simulink model "Pt_Engine_TC_CS8"  (Simulink 7.0)
settings: Solver=ode45  StartTime=0  StopTime=20  FixedStep=TSTEP  RelTol=1e-3
PreLoadFcn:
  | cd extensions\simulink\pt_engine_tc
  | mengine_carpet_eclass
  | torq_conv_map_eclass
  | Run_ft4wd_eclass
  | cd ..\..\..
undefined symbols (not defined in the file): AV_ENG_IDLE, IENG, INV_CAP_TC_TABLE, ITC_INPUT_SHAFT, MENGINE_CARPET, RM_TC_TABLE
libraries: Solver_SF x1
settings Model: Creator=dhall  LastModifiedBy=ywata  ExtModeTrigMode=oneshot  ExtModeArmWhenConnect=off
settings DataIOCC: LimitDataPoints=off  SaveOutput=off  SaveTime=off  SignalLoggingName=sigsOut
settings OptimizationCC: BooleanDataType=off
settings DebuggingCC: SaveWithParameterizedLinksMsg=none  SignalResolutionControl=TryResolveAllWithWarning  SolverPrmCheckMsg=none  MultiTaskDSMMsg=warning  MultiTaskCondExecSysMsg=none  StrictBusMsg=None
settings HardwareCC: TargetUnknown=on
settings RTWCC: IncludeERTFirstTime=on
settings GRTTargetCC: TargetFcnLib=ansi_tfl_tmw.mat  ModelReferenceCompliant=off  MatFileLogging=off

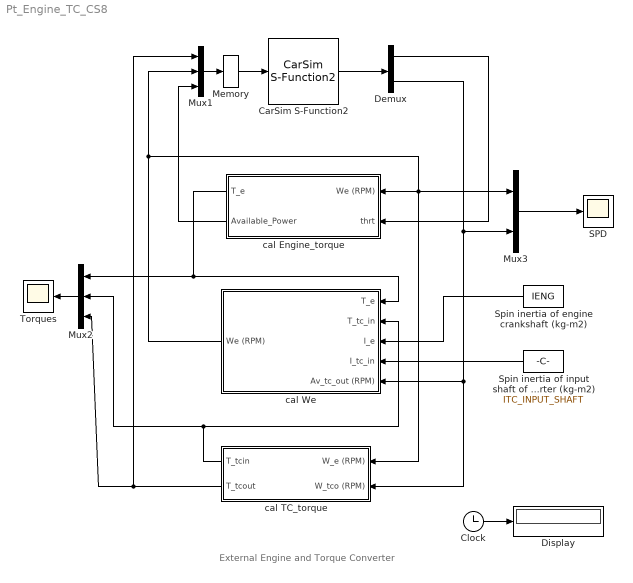
== system Pt_Engine_TC_CS8 ==
  note: External Engine and Torque Converter
  CarSim S-Function2 : Solver_SF/CarSim S-Function2  Priority=1  VehicleCode=???
      settings: AttributesFormatString=Vehicle Code: %<VehicleCode>
  Clock : Clock
      settings: Decimation=10
  Demux : Demux  Outputs=2
  Display : Display
  Memory : Memory
  Mux1 : Mux  Inputs=3
  Mux2 : Mux  Orientation=left  Inputs=3
  Mux3 : Mux  Inputs=2
  SPD : Scope
      settings: TimeRange=20  YMin=0  YMax=4500
  Spin inertia of engine crankshaft (kg-m2) : Constant  Orientation=left  Value=IENG  OutDataType=sfix(16)  OutScaling=2^0
  Spin inertia of input shaft of torque converter (kg-m2) : Constant  Orientation=left  Value=ITC_INPUT_SHAFT  OutDataType=sfix(16)  OutScaling=2^0
  Torques : Scope
      settings: TimeRange=20  YMin=-50  YMax=600
  cal Engine_torque : Subsystem  Orientation=left
  cal TC_torque : Subsystem  Orientation=left
  cal We : Subsystem  Orientation=left
  wires:
  cal We/1(We (RPM)) -> cal TC_torque/1(W_e (RPM)), Mux3/1, cal Engine_torque/1(We (RPM)), Mux1/2
  Spin inertia of engine crankshaft (kg-m2)/1 -> cal We/3(I_e)
  Spin inertia of input shaft of torque converter (kg-m2)/1 -> cal We/4(I_tc_in)
  cal Engine_torque/1(T_e) -> Mux2/1, cal We/1(T_e)
  cal TC_torque/1(T_tcin) -> Mux2/2, cal We/2(T_tc_in)
  CarSim S-Function2/1 -> Demux/1
  Demux/1 -> cal Engine_torque/2(thrt)
  Demux/2 -> cal TC_torque/2(W_tco (RPM)), cal We/5(Av_tc_out (RPM)), Mux3/2
  cal TC_torque/2(T_tcout) -> Mux2/3, Mux1/1
  Mux2/1 -> Torques/1
  Mux3/1 -> SPD/1
  Clock/1 -> Display/1
  cal Engine_torque/2(Available_Power) -> Mux1/3
  Mux1/1 -> Memory/1
  Memory/1 -> CarSim S-Function2/1

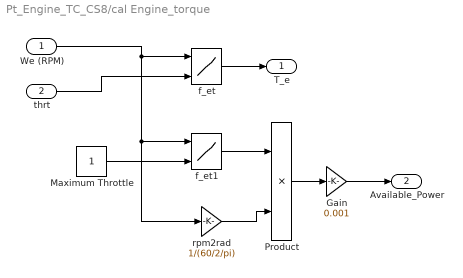
== system Pt_Engine_TC_CS8/cal Engine_torque ==
  We (RPM) : Inport  OutDataType=sfix(16)  OutScaling=2^0
  thrt : Inport  Port=2  OutDataType=sfix(16)  OutScaling=2^0
  Gain : Gain  Gain=0.001  ParameterDataType=sfix(16)  ParameterScaling=2^0  OutDataType=sfix(16)  OutScaling=2^0  SaturateOnIntegerOverflow=on
  Maximum Throttle : Constant  OutDataType=sfix(16)  OutScaling=2^0
  Product : Product  OutDataType=sfix(16)  OutScaling=2^0  SaturateOnIntegerOverflow=on  InputSameDT=on
  f_et : Lookup2D  RowIndex=MENGINE_CARPET(2:19,1)  ColumnIndex=MENGINE_CARPET(1,2:11)  Table=MENGINE_CARPET(2:19,2:11)  OutDataType=sfix(16)  OutScaling=2^0  SaturateOnIntegerOverflow=on  InputSameDT=on
  f_et1 : Lookup2D  RowIndex=MENGINE_CARPET(2:19,1)  ColumnIndex=MENGINE_CARPET(1,2:11)  Table=MENGINE_CARPET(2:19,2:11)  OutDataType=sfix(16)  OutScaling=2^0  SaturateOnIntegerOverflow=on  InputSameDT=on
  rpm2rad : Gain  Gain=1/(60/2/pi)  ParameterDataType=sfix(16)  ParameterScaling=2^0  OutDataType=sfix(16)  OutScaling=2^0  SaturateOnIntegerOverflow=on
  T_e : Outport
  Available_Power : Outport  Port=2
  wires:
  We (RPM)/1 -> f_et/1, rpm2rad/1, f_et1/1
  f_et/1 -> T_e/1
  thrt/1 -> f_et/2
  Maximum Throttle/1 -> f_et1/2
  f_et1/1 -> Product/1
  rpm2rad/1 -> Product/2
  Product/1 -> Gain/1
  Gain/1 -> Available_Power/1

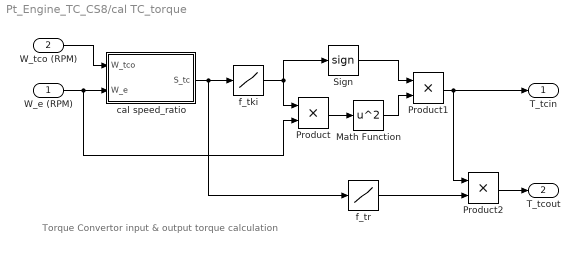
== system Pt_Engine_TC_CS8/cal TC_torque ==
  note: Torque Convertor input & output torque calculation
  W_e (RPM) : Inport  OutDataType=sfix(16)  OutScaling=2^0
  W_tco (RPM) : Inport  Port=2  OutDataType=sfix(16)  OutScaling=2^0
  Math Function : Math  Operator=square  SaturateOnIntegerOverflow=on
  Product : Product  OutDataType=sfix(16)  OutScaling=2^0  SaturateOnIntegerOverflow=on  InputSameDT=on
  Product1 : Product  OutDataType=sfix(16)  OutScaling=2^0  SaturateOnIntegerOverflow=on  InputSameDT=on
  Product2 : Product  OutDataType=sfix(16)  OutScaling=2^0  SaturateOnIntegerOverflow=on  InputSameDT=on
  Sign : Signum
  cal speed_ratio : Subsystem
  f_tki : Lookup  InputValues=INV_CAP_TC_TABLE(:,1)  Table=INV_CAP_TC_TABLE(:,2)  OutDataType=sfix(16)  OutScaling=2^0  SaturateOnIntegerOverflow=on
  f_tr : Lookup  InputValues=RM_TC_TABLE(:,1)  Table=RM_TC_TABLE(:,2)  OutDataType=sfix(16)  OutScaling=2^0  SaturateOnIntegerOverflow=on
  T_tcin : Outport
  T_tcout : Outport  Port=2
  wires:
  Product/1 -> Math Function/1
  f_tki/1 -> Product/1, Sign/1
  Math Function/1 -> Product1/2
  Sign/1 -> Product1/1
  W_e (RPM)/1 -> cal speed_ratio/2(W_e), Product/2
  cal speed_ratio/1(S_tc) -> f_tki/1, f_tr/1
  f_tr/1 -> Product2/2
  Product1/1 -> Product2/1, T_tcin/1
  W_tco (RPM)/1 -> cal speed_ratio/1(W_tco)
  Product2/1 -> T_tcout/1

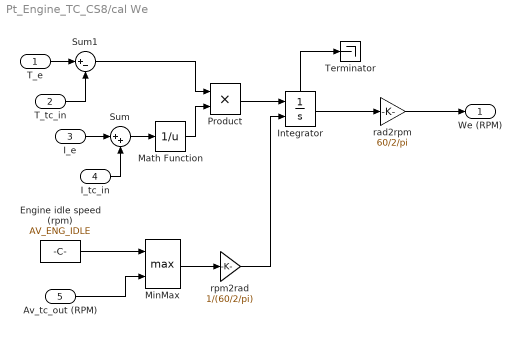
== system Pt_Engine_TC_CS8/cal We ==
  T_e : Inport  OutDataType=sfix(16)  OutScaling=2^0
  T_tc_in : Inport  Port=2  OutDataType=sfix(16)  OutScaling=2^0
  I_e : Inport  Port=3  OutDataType=sfix(16)  OutScaling=2^0
  I_tc_in : Inport  Port=4  OutDataType=sfix(16)  OutScaling=2^0
  Av_tc_out (RPM) : Inport  Port=5  OutDataType=sfix(16)  OutScaling=2^0
  Engine idle speed (rpm) : Constant  Value=AV_ENG_IDLE  OutDataType=sfix(16)  OutScaling=2^0
  Integrator : Integrator  InitialConditionSource=external  InitialCondition=AV_ENG_IDLE*2*pi/60  ShowStatePort=on
  Math Function : Math  Operator=reciprocal  SaturateOnIntegerOverflow=on
  MinMax : MinMax  Function=max  Inputs=2  SaturateOnIntegerOverflow=on  InputSameDT=on
  Product : Product  OutDataType=sfix(16)  OutScaling=2^0  SaturateOnIntegerOverflow=on  InputSameDT=on
  Sum : Sum  Inputs=|++  OutDataType=sfix(16)  OutScaling=2^0  SaturateOnIntegerOverflow=on  InputSameDT=on
  Sum1 : Sum  Inputs=|+-  OutDataType=sfix(16)  OutScaling=2^0  SaturateOnIntegerOverflow=on  InputSameDT=on
  Terminator : Terminator
  rad2rpm : Gain  Gain=60/2/pi  ParameterDataType=sfix(16)  ParameterScaling=2^0  OutDataType=sfix(16)  OutScaling=2^0  SaturateOnIntegerOverflow=on
  rpm2rad : Gain  Gain=1/(60/2/pi)  ParameterDataType=sfix(16)  ParameterScaling=2^0  OutDataType=sfix(16)  OutScaling=2^0  SaturateOnIntegerOverflow=on
  We (RPM) : Outport
  wires:
  Integrator/State -> Terminator/1
  rpm2rad/1 -> Integrator/2
  Integrator/1 -> rad2rpm/1
  Product/1 -> Integrator/1
  I_tc_in/1 -> Sum/2
  I_e/1 -> Sum/1
  T_tc_in/1 -> Sum1/2
  Sum/1 -> Math Function/1
  T_e/1 -> Sum1/1
  Sum1/1 -> Product/1
  Math Function/1 -> Product/2
  rad2rpm/1 -> We (RPM)/1
  Engine idle speed (rpm)/1 -> MinMax/1
  Av_tc_out (RPM)/1 -> MinMax/2
  MinMax/1 -> rpm2rad/1

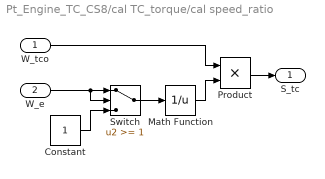
== system Pt_Engine_TC_CS8/cal TC_torque/cal speed_ratio ==
  W_tco : Inport  OutDataType=sfix(16)  OutScaling=2^0
  W_e : Inport  Port=2  OutDataType=sfix(16)  OutScaling=2^0
  Constant : Constant  OutDataType=sfix(16)  OutScaling=2^0
  Math Function : Math  Operator=reciprocal  SaturateOnIntegerOverflow=on
  Product : Product  OutDataType=sfix(16)  OutScaling=2^0  SaturateOnIntegerOverflow=on  InputSameDT=on
  Switch : Switch  Threshold=1  SaturateOnIntegerOverflow=on  InputSameDT=on
  S_tc : Outport
  wires:
  Math Function/1 -> Product/2
  W_tco/1 -> Product/1
  Product/1 -> S_tc/1
  Switch/1 -> Math Function/1
  W_e/1 -> Switch/1, Switch/2
  Constant/1 -> Switch/3
